simulink model "FOC_sensored"  (R2026a)
settings: Solver=VariableStepAuto  StopTime=0.5  MaxStep=1e-4  RelTol=1e-4
values from neighbouring files (symbols this model uses):
  Encoder_resolution = 4000    [FOC_sensored_script.m]
  In = 1    [FOC_sensored_script.m]
  J = 0.1e-4    (= 1e-05)    [FOC_sensored_script.m]
  Kr_cont_current = (2*omega_n*tau_q*zeta - 1) / K_q    [FOC_sensored_script.m]
  Kr_cont_speed = (2*omega_n_speed*tau_w*zeta_speed - 1) / K_w    [FOC_sensored_script.m]
  Kr_direct_back_current = (1-delta2*exp(Ts_current/tau_q)) / (K_q*(exp(Ts_current/tau_q)-1))    [FOC_sensored_script.m]
  Kr_direct_back_speed = (1-delta2*exp(Ts_speed/tau_w)) / (K_w*(exp(Ts_speed/tau_w)-1))    [FOC_sensored_script.m]
  Kr_direct_forw_current = (1+(1+delta1)*exp(Ts_current/tau_q)) / (K_q*(exp(Ts_current/tau_q)-1))    [FOC_sensored_script.m]
  Kr_direct_tustin_current = (2-exp(Ts_current/tau_q)*(delta2-delta1-1)) / (2*K_q*(exp(Ts_current/tau_q)-1))    [FOC_sensored_script.m]
  Kr_direct_tustin_speed = (2-exp(Ts_speed/tau_w)*(delta2-delta1-1)) / (2*K_w*(exp(Ts_speed/tau_w)-1))    [FOC_sensored_script.m]
  Ls = 330e-6/2    (= 0.000165)    [FOC_sensored_script.m]
  Mn = Pn/wn    [FOC_sensored_script.m]
  nn = ns/pp    (= 6000)    [FOC_sensored_script.m]
  pp = (60*fs)/ns    (= 4)    [FOC_sensored_script.m]
  Psir = 0.0064    [FOC_sensored_script.m]
  T_speed_feedback = 0.0005    [FOC_sensored_script.m]
  Ti_cont_current = (2*omega_n*tau_q*zeta - 1) / (tau_q * omega_n^2)    [FOC_sensored_script.m]
  Ti_cont_speed = (2*omega_n_speed*tau_w*zeta_speed - 1) / (tau_w * omega_n_speed^2)    [FOC_sensored_script.m]
  Ti_direct_back_current = Ts_current * (exp(-Ts_current/tau_q)-delta2) / (1+delta1+delta2)    [FOC_sensored_script.m]
  Ti_direct_back_speed = Ts_speed * (exp(-Ts_speed/tau_w)-delta2) / (1+delta1+delta2)    [FOC_sensored_script.m]
  Ti_direct_forw_current = Ts_current * (1+delta1+exp(-Ts_current/tau_q)) / (1+delta1+delta2)    [FOC_sensored_script.m]
  Ti_direct_forw_speed = Ts_speed * (1+delta1+exp(-Ts_speed/tau_w)) / (1+delta1+delta2)    [FOC_sensored_script.m]
  Ti_direct_tustin_current = Ts_current*(2*exp(-Ts_current/tau_q)+delta1-delta2+1) / (2*(1+delta1+delta2))    [FOC_sensored_script.m]
  Ti_direct_tustin_speed = Ts_speed*(2*exp(-Ts_speed/tau_w)+delta1-delta2+1) / (2*(1+delta1+delta2))    [FOC_sensored_script.m]
  Ts_current = 100e-6    (= 0.0001)    [FOC_sensored_script.m]
  Udc = 24    [FOC_sensored_script.m]
undefined symbols (not defined in the file or in its folder): Ld, Lq
libraries: fl_lib x48, nesl_utility x42, ee_lib x18, eeTransforms x12
(part 2 of 3)

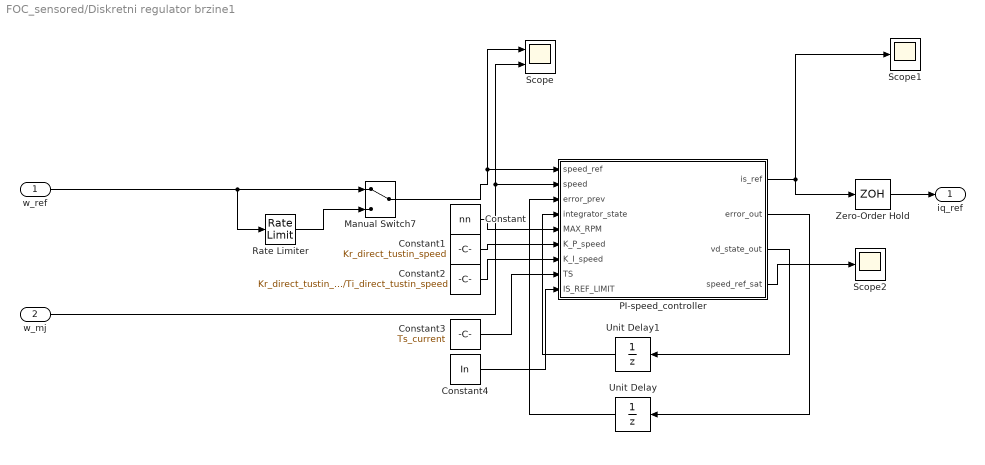
== system FOC_sensored/Diskretni regulator brzine1 ==
  w_ref : Inport
  w_mj : Inport  Port=2
  Constant : Constant  Value=nn  SampleTime=Ts_current
  Constant1 : Constant  Value=Kr_direct_tustin_speed  SampleTime=Ts_current
  Constant2 : Constant  Value=Kr_direct_tustin_speed/Ti_direct_tustin_speed  SampleTime=Ts_current
  Constant3 : Constant  Value=Ts_current  SampleTime=Ts_current
  Constant4 : Constant  Value=In  SampleTime=Ts_current
  Manual Switch7 : ManualSwitch
  PI-speed_controller : MATLAB Function  TreatAsAtomicUnit=on
  Rate Limiter : RateLimiter  RisingSlewLimit=Mn/J  FallingSlewLimit=-Mn/J  SampleTimeMode=inherited
  Scope : Scope  NumInputPorts=2
      settings: ActiveDisplayYMinimum=-62.500309400179823  ActiveDisplayYMaximum=562.50278460161849  DataLoggingVariableName=ScopeData4
  Scope1 : Scope
      settings: ActiveDisplayYMinimum=-62.5113191756852  ActiveDisplayYMaximum=70.802739564965421  DataLoggingVariableName=ScopeData5
  Scope2 : Scope
      settings: ActiveDisplayYMinimum=-1  ActiveDisplayYMaximum=1  DataLoggingVariableName=ScopeData10
  Unit Delay : UnitDelay  SampleTime=Ts_current
  Unit Delay1 : UnitDelay  SampleTime=Ts_current
  Zero-Order Hold : ZeroOrderHold  SampleTime=Ts_current
  iq_ref : Outport
  wires:
  Rate Limiter/1 -> Manual Switch7/2
  PI-speed_controller/2(error_out) -> Unit Delay/1
  Unit Delay/1 -> PI-speed_controller/3(error_prev)
  PI-speed_controller/3(vd_state_out) -> Unit Delay1/1
  Unit Delay1/1 -> PI-speed_controller/4(integrator_state)
  w_ref/1 -> Manual Switch7/1, Rate Limiter/1
  Manual Switch7/1 -> Scope/1, PI-speed_controller/1(speed_ref)
  w_mj/1 -> Scope/2, PI-speed_controller/2(speed)
  PI-speed_controller/1(is_ref) -> Scope1/1, Zero-Order Hold/1
  PI-speed_controller/4(speed_ref_sat) -> Scope2/1
  Zero-Order Hold/1 -> iq_ref/1
  Constant/1 -> PI-speed_controller/5(MAX_RPM)
  Constant1/1 -> PI-speed_controller/6(K_P_speed)
  Constant2/1 -> PI-speed_controller/7(K_I_speed)
  Constant3/1 -> PI-speed_controller/8(TS)
  Constant4/1 -> PI-speed_controller/9(IS_REF_LIMIT)

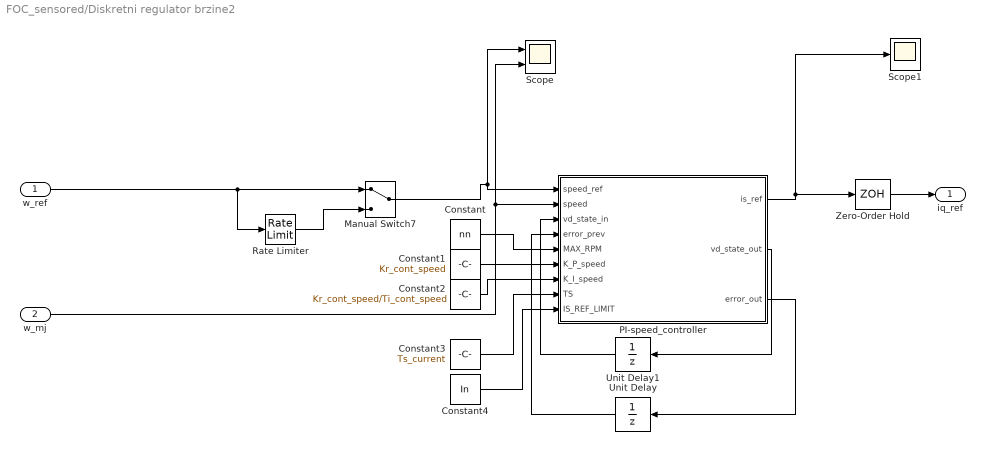
== system FOC_sensored/Diskretni regulator brzine2 ==
  w_ref : Inport
  w_mj : Inport  Port=2
  Constant : Constant  Value=nn  SampleTime=Ts_current
  Constant1 : Constant  Value=Kr_cont_speed  SampleTime=Ts_current
  Constant2 : Constant  Value=Kr_cont_speed/Ti_cont_speed  SampleTime=Ts_current
  Constant3 : Constant  Value=Ts_current  SampleTime=Ts_current
  Constant4 : Constant  Value=In  SampleTime=Ts_current
  Manual Switch7 : ManualSwitch
  PI-speed_controller : MATLAB Function  TreatAsAtomicUnit=on
  Rate Limiter : RateLimiter  RisingSlewLimit=Mn/J  FallingSlewLimit=-Mn/J  SampleTimeMode=inherited
  Scope : Scope  NumInputPorts=2
      settings: ActiveDisplayYMinimum=-62.500309400179823  ActiveDisplayYMaximum=562.50278460161849  DataLoggingVariableName=ScopeData4
  Scope1 : Scope
      settings: ActiveDisplayYMinimum=-62.5113191756852  ActiveDisplayYMaximum=70.802739564965421  DataLoggingVariableName=ScopeData5
  Unit Delay : UnitDelay  SampleTime=Ts_current
  Unit Delay1 : UnitDelay  SampleTime=Ts_current
  Zero-Order Hold : ZeroOrderHold  SampleTime=Ts_current
  iq_ref : Outport
  wires:
  Rate Limiter/1 -> Manual Switch7/2
  PI-speed_controller/3(error_out) -> Unit Delay/1
  Unit Delay/1 -> PI-speed_controller/4(error_prev)
  PI-speed_controller/2(vd_state_out) -> Unit Delay1/1
  Unit Delay1/1 -> PI-speed_controller/3(vd_state_in)
  w_ref/1 -> Manual Switch7/1, Rate Limiter/1
  Manual Switch7/1 -> Scope/1, PI-speed_controller/1(speed_ref)
  w_mj/1 -> Scope/2, PI-speed_controller/2(speed)
  PI-speed_controller/1(is_ref) -> Scope1/1, Zero-Order Hold/1
  Zero-Order Hold/1 -> iq_ref/1
  Constant/1 -> PI-speed_controller/5(MAX_RPM)
  Constant1/1 -> PI-speed_controller/6(K_P_speed)
  Constant2/1 -> PI-speed_controller/7(K_I_speed)
  Constant3/1 -> PI-speed_controller/8(TS)
  Constant4/1 -> PI-speed_controller/9(IS_REF_LIMIT)

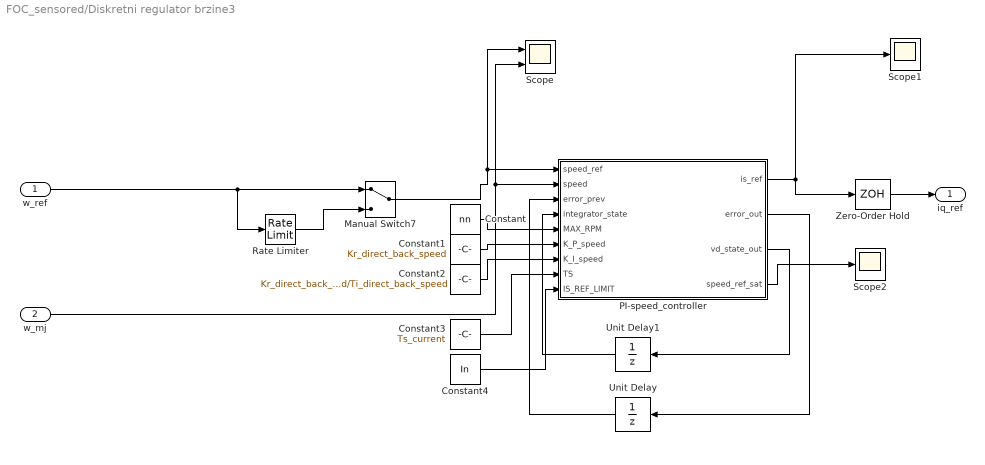
== system FOC_sensored/Diskretni regulator brzine3 ==
  w_ref : Inport
  w_mj : Inport  Port=2
  Constant : Constant  Value=nn  SampleTime=Ts_current
  Constant1 : Constant  Value=Kr_direct_back_speed  SampleTime=Ts_current
  Constant2 : Constant  Value=Kr_direct_back_speed/Ti_direct_back_speed  SampleTime=Ts_current
  Constant3 : Constant  Value=Ts_current  SampleTime=Ts_current
  Constant4 : Constant  Value=In  SampleTime=Ts_current
  Manual Switch7 : ManualSwitch
  PI-speed_controller : MATLAB Function  TreatAsAtomicUnit=on
  Rate Limiter : RateLimiter  RisingSlewLimit=Mn/J  FallingSlewLimit=-Mn/J  SampleTimeMode=inherited
  Scope : Scope  NumInputPorts=2
      settings: ActiveDisplayYMinimum=-62.500309400179823  ActiveDisplayYMaximum=562.50278460161849  DataLoggingVariableName=ScopeData4
  Scope1 : Scope
      settings: ActiveDisplayYMinimum=-62.5113191756852  ActiveDisplayYMaximum=70.802739564965421  DataLoggingVariableName=ScopeData5
  Scope2 : Scope
      settings: ActiveDisplayYMinimum=-1  ActiveDisplayYMaximum=1  DataLoggingVariableName=ScopeData10
  Unit Delay : UnitDelay  SampleTime=Ts_current
  Unit Delay1 : UnitDelay  SampleTime=Ts_current
  Zero-Order Hold : ZeroOrderHold  SampleTime=Ts_current
  iq_ref : Outport
  wires:
  Rate Limiter/1 -> Manual Switch7/2
  PI-speed_controller/2(error_out) -> Unit Delay/1
  Unit Delay/1 -> PI-speed_controller/3(error_prev)
  PI-speed_controller/3(vd_state_out) -> Unit Delay1/1
  Unit Delay1/1 -> PI-speed_controller/4(integrator_state)
  w_ref/1 -> Manual Switch7/1, Rate Limiter/1
  Manual Switch7/1 -> Scope/1, PI-speed_controller/1(speed_ref)
  w_mj/1 -> Scope/2, PI-speed_controller/2(speed)
  PI-speed_controller/1(is_ref) -> Scope1/1, Zero-Order Hold/1
  PI-speed_controller/4(speed_ref_sat) -> Scope2/1
  Zero-Order Hold/1 -> iq_ref/1
  Constant/1 -> PI-speed_controller/5(MAX_RPM)
  Constant1/1 -> PI-speed_controller/6(K_P_speed)
  Constant2/1 -> PI-speed_controller/7(K_I_speed)
  Constant3/1 -> PI-speed_controller/8(TS)
  Constant4/1 -> PI-speed_controller/9(IS_REF_LIMIT)

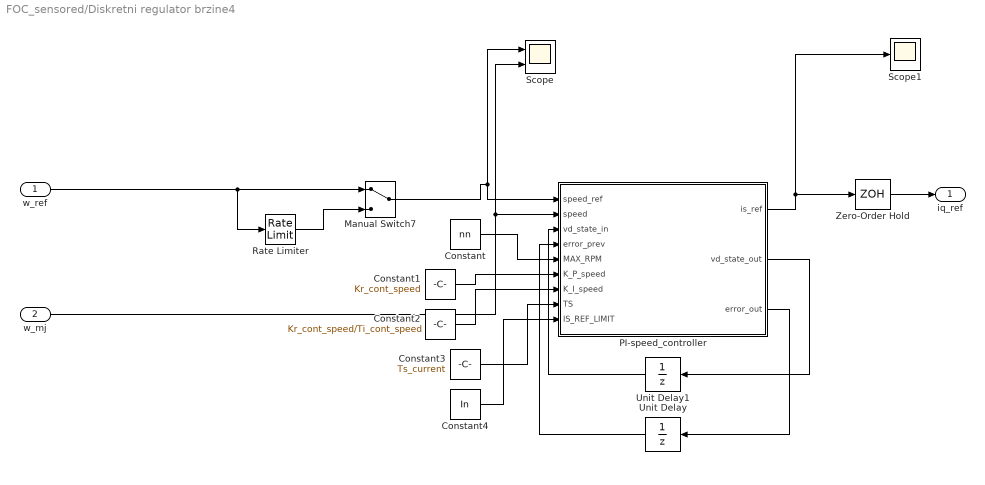
== system FOC_sensored/Diskretni regulator brzine4 ==
  w_ref : Inport
  w_mj : Inport  Port=2
  Constant : Constant  Value=nn  SampleTime=Ts_current
  Constant1 : Constant  Value=Kr_cont_speed  SampleTime=Ts_current
  Constant2 : Constant  Value=Kr_cont_speed/Ti_cont_speed  SampleTime=Ts_current
  Constant3 : Constant  Value=Ts_current  SampleTime=Ts_current
  Constant4 : Constant  Value=In  SampleTime=Ts_current
  Manual Switch7 : ManualSwitch
  PI-speed_controller : MATLAB Function  TreatAsAtomicUnit=on
  Rate Limiter : RateLimiter  RisingSlewLimit=Mn/J  FallingSlewLimit=-Mn/J  SampleTimeMode=inherited
  Scope : Scope  NumInputPorts=2
      settings: ActiveDisplayYMinimum=-62.500309400179823  ActiveDisplayYMaximum=562.50278460161849  DataLoggingVariableName=ScopeData4
  Scope1 : Scope
      settings: ActiveDisplayYMinimum=-62.5113191756852  ActiveDisplayYMaximum=70.802739564965421  DataLoggingVariableName=ScopeData5
  Unit Delay : UnitDelay  SampleTime=Ts_current
  Unit Delay1 : UnitDelay  SampleTime=Ts_current
  Zero-Order Hold : ZeroOrderHold  SampleTime=Ts_current
  iq_ref : Outport
  wires:
  Rate Limiter/1 -> Manual Switch7/2
  PI-speed_controller/3(error_out) -> Unit Delay/1
  Unit Delay/1 -> PI-speed_controller/4(error_prev)
  PI-speed_controller/2(vd_state_out) -> Unit Delay1/1
  Unit Delay1/1 -> PI-speed_controller/3(vd_state_in)
  w_ref/1 -> Manual Switch7/1, Rate Limiter/1
  Manual Switch7/1 -> Scope/1, PI-speed_controller/1(speed_ref)
  w_mj/1 -> Scope/2, PI-speed_controller/2(speed)
  PI-speed_controller/1(is_ref) -> Scope1/1, Zero-Order Hold/1
  Zero-Order Hold/1 -> iq_ref/1
  Constant/1 -> PI-speed_controller/5(MAX_RPM)
  Constant1/1 -> PI-speed_controller/6(K_P_speed)
  Constant2/1 -> PI-speed_controller/7(K_I_speed)
  Constant3/1 -> PI-speed_controller/8(TS)
  Constant4/1 -> PI-speed_controller/9(IS_REF_LIMIT)

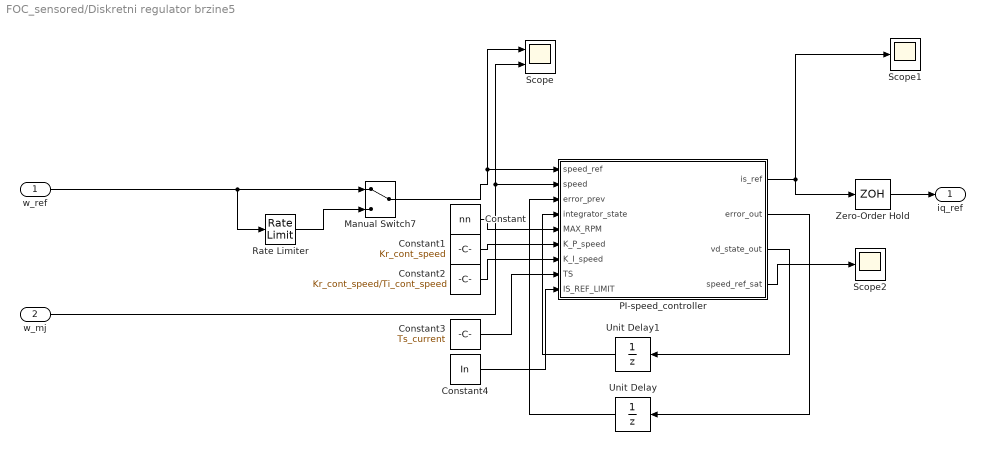
== system FOC_sensored/Diskretni regulator brzine5 ==
  w_ref : Inport
  w_mj : Inport  Port=2
  Constant : Constant  Value=nn  SampleTime=Ts_current
  Constant1 : Constant  Value=Kr_cont_speed  SampleTime=Ts_current
  Constant2 : Constant  Value=Kr_cont_speed/Ti_cont_speed  SampleTime=Ts_current
  Constant3 : Constant  Value=Ts_current  SampleTime=Ts_current
  Constant4 : Constant  Value=In  SampleTime=Ts_current
  Manual Switch7 : ManualSwitch
  PI-speed_controller : MATLAB Function  TreatAsAtomicUnit=on
  Rate Limiter : RateLimiter  RisingSlewLimit=Mn/J  FallingSlewLimit=-Mn/J  SampleTimeMode=inherited
  Scope : Scope  NumInputPorts=2
      settings: ActiveDisplayYMinimum=-62.500309400179823  ActiveDisplayYMaximum=562.50278460161849  DataLoggingVariableName=ScopeData4
  Scope1 : Scope
      settings: ActiveDisplayYMinimum=-62.5113191756852  ActiveDisplayYMaximum=70.802739564965421  DataLoggingVariableName=ScopeData5
  Scope2 : Scope
      settings: ActiveDisplayYMinimum=-1  ActiveDisplayYMaximum=1  DataLoggingVariableName=ScopeData10
  Unit Delay : UnitDelay  SampleTime=Ts_current
  Unit Delay1 : UnitDelay  SampleTime=Ts_current
  Zero-Order Hold : ZeroOrderHold  SampleTime=Ts_current
  iq_ref : Outport
  wires:
  Rate Limiter/1 -> Manual Switch7/2
  PI-speed_controller/2(error_out) -> Unit Delay/1
  Unit Delay/1 -> PI-speed_controller/3(error_prev)
  PI-speed_controller/3(vd_state_out) -> Unit Delay1/1
  Unit Delay1/1 -> PI-speed_controller/4(integrator_state)
  w_ref/1 -> Manual Switch7/1, Rate Limiter/1
  Manual Switch7/1 -> Scope/1, PI-speed_controller/1(speed_ref)
  w_mj/1 -> Scope/2, PI-speed_controller/2(speed)
  PI-speed_controller/1(is_ref) -> Scope1/1, Zero-Order Hold/1
  PI-speed_controller/4(speed_ref_sat) -> Scope2/1
  Zero-Order Hold/1 -> iq_ref/1
  Constant/1 -> PI-speed_controller/5(MAX_RPM)
  Constant1/1 -> PI-speed_controller/6(K_P_speed)
  Constant2/1 -> PI-speed_controller/7(K_I_speed)
  Constant3/1 -> PI-speed_controller/8(TS)
  Constant4/1 -> PI-speed_controller/9(IS_REF_LIMIT)

== system FOC_sensored/Diskretni regulator brzine6 ==
  w_ref : Inport
  w_mj : Inport  Port=2
  Constant : Constant  Value=nn  SampleTime=Ts_current
  Constant1 : Constant  Value=Kr_cont_speed  SampleTime=Ts_current
  Constant2 : Constant  Value=Kr_cont_speed/Ti_cont_speed  SampleTime=Ts_current
  Constant3 : Constant  Value=Ts_current  SampleTime=Ts_current
  Constant4 : Constant  Value=In  SampleTime=Ts_current
  Manual Switch7 : ManualSwitch
  PI-speed_controller : MATLAB Function  TreatAsAtomicUnit=on
  Rate Limiter : RateLimiter  RisingSlewLimit=Mn/J  FallingSlewLimit=-Mn/J  SampleTimeMode=inherited
  Scope : Scope  NumInputPorts=2
      settings: ActiveDisplayYMinimum=-62.500309400179823  ActiveDisplayYMaximum=562.50278460161849  DataLoggingVariableName=ScopeData4
  Scope1 : Scope
      settings: ActiveDisplayYMinimum=-62.5113191756852  ActiveDisplayYMaximum=70.802739564965421  DataLoggingVariableName=ScopeData5
  Unit Delay : UnitDelay  SampleTime=Ts_current
  Unit Delay1 : UnitDelay  SampleTime=Ts_current
  Zero-Order Hold : ZeroOrderHold  SampleTime=Ts_current
  iq_ref : Outport
  wires:
  Rate Limiter/1 -> Manual Switch7/2
  PI-speed_controller/3(error_out) -> Unit Delay/1
  Unit Delay/1 -> PI-speed_controller/4(error_prev)
  PI-speed_controller/2(vd_state_out) -> Unit Delay1/1
  Unit Delay1/1 -> PI-speed_controller/3(vd_state_in)
  w_ref/1 -> Manual Switch7/1, Rate Limiter/1
  Manual Switch7/1 -> Scope/1, PI-speed_controller/1(speed_ref)
  w_mj/1 -> Scope/2, PI-speed_controller/2(speed)
  PI-speed_controller/1(is_ref) -> Scope1/1, Zero-Order Hold/1
  Zero-Order Hold/1 -> iq_ref/1
  Constant/1 -> PI-speed_controller/5(MAX_RPM)
  Constant1/1 -> PI-speed_controller/6(K_P_speed)
  Constant2/1 -> PI-speed_controller/7(K_I_speed)
  Constant3/1 -> PI-speed_controller/8(TS)
  Constant4/1 -> PI-speed_controller/9(IS_REF_LIMIT)

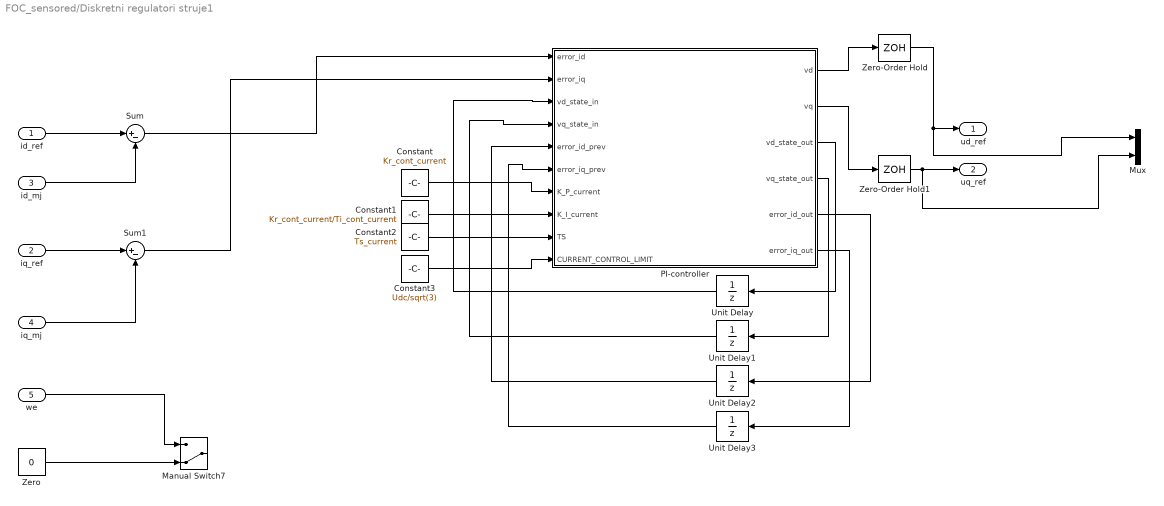
== system FOC_sensored/Diskretni regulatori struje1 ==
  id_ref : Inport
  iq_ref : Inport  Port=2
  id_mj : Inport  Port=3
  iq_mj : Inport  Port=4
  we : Inport  Port=5
  Constant : Constant  Value=Kr_cont_current  SampleTime=Ts_current
  Constant1 : Constant  Value=Kr_cont_current/Ti_cont_current  SampleTime=Ts_current
  Constant2 : Constant  Value=Ts_current  SampleTime=Ts_current
  Constant3 : Constant  Value=Udc/sqrt(3)  SampleTime=Ts_current
  Manual Switch7 : ManualSwitch  CurrentSetting=0
  Mux : Mux  Inputs=2
  PI-controller : MATLAB Function  TreatAsAtomicUnit=on
  Sum : Sum  Inputs=|+-
  Sum1 : Sum  Inputs=|+-
  Unit Delay{,1..3} (4 alike) : UnitDelay  SampleTime=Ts_current
  Zero : Constant  Value=0  OutDataTypeStr=Inherit: Inherit via back propagation
  Zero-Order Hold : ZeroOrderHold  SampleTime=Ts_current
  Zero-Order Hold1 : ZeroOrderHold  SampleTime=Ts_current
  ud_ref : Outport
  uq_ref : Outport  Port=2
  wires:
  id_ref/1 -> Sum/1
  iq_ref/1 -> Sum1/1
  Sum/1 -> PI-controller/1(error_id)
  id_mj/1 -> Sum/2
  iq_mj/1 -> Sum1/2
  PI-controller/3(vd_state_out) -> Unit Delay/1
  PI-controller/4(vq_state_out) -> Unit Delay1/1
  PI-controller/1(vd) -> Zero-Order Hold/1
  PI-controller/2(vq) -> Zero-Order Hold1/1
  Zero-Order Hold/1 -> Mux/1, ud_ref/1
  Zero-Order Hold1/1 -> Mux/2, uq_ref/1
  Zero/1 -> Manual Switch7/2
  we/1 -> Manual Switch7/1
  Sum1/1 -> PI-controller/2(error_iq)
  Unit Delay/1 -> PI-controller/3(vd_state_in)
  Unit Delay1/1 -> PI-controller/4(vq_state_in)
  PI-controller/5(error_id_out) -> Unit Delay2/1
  Unit Delay2/1 -> PI-controller/5(error_id_prev)
  PI-controller/6(error_iq_out) -> Unit Delay3/1
  Unit Delay3/1 -> PI-controller/6(error_iq_prev)
  Constant/1 -> PI-controller/7(K_P_current)
  Constant1/1 -> PI-controller/8(K_I_current)
  Constant2/1 -> PI-controller/9(TS)
  Constant3/1 -> PI-controller/10(CURRENT_CONTROL_LIMIT)

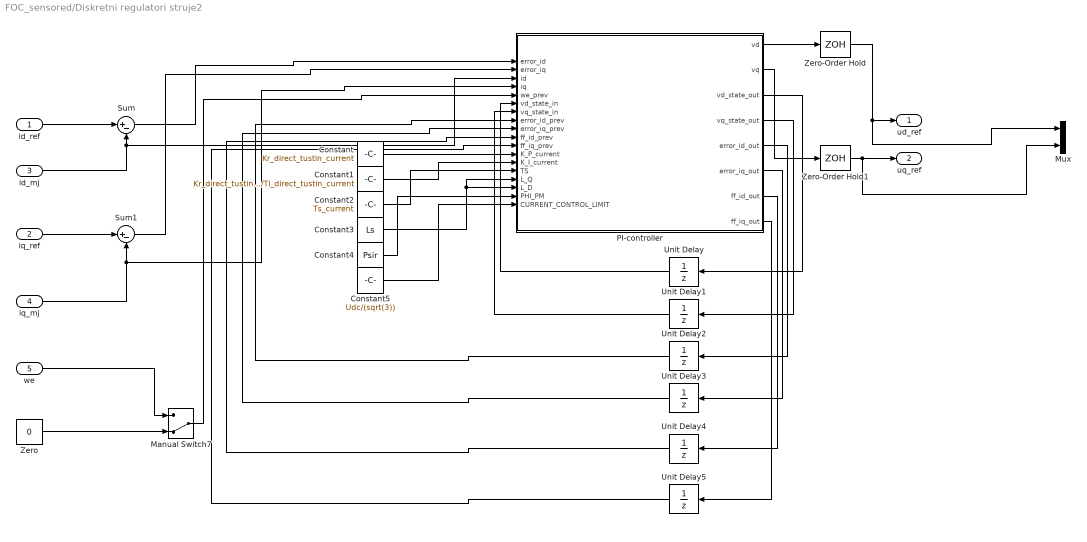
== system FOC_sensored/Diskretni regulatori struje2 ==
  id_ref : Inport
  iq_ref : Inport  Port=2
  id_mj : Inport  Port=3
  iq_mj : Inport  Port=4
  we : Inport  Port=5
  Constant : Constant  Value=Kr_direct_tustin_current  SampleTime=Ts_current
  Constant1 : Constant  Value=Kr_direct_tustin_current/Ti_direct_tustin_current  SampleTime=Ts_current
  Constant2 : Constant  Value=Ts_current  SampleTime=Ts_current
  Constant3 : Constant  Value=Ls  SampleTime=Ts_current
  Constant4 : Constant  Value=Psir  SampleTime=Ts_current
  Constant5 : Constant  Value=Udc/(sqrt(3))  SampleTime=Ts_current
  Manual Switch7 : ManualSwitch  CurrentSetting=0
  Mux : Mux  Inputs=2
  PI-controller : MATLAB Function  TreatAsAtomicUnit=on
  Sum : Sum  Inputs=|+-
  Sum1 : Sum  Inputs=|+-
  Unit Delay{,1..5} (6 alike) : UnitDelay  SampleTime=Ts_current
  Zero : Constant  Value=0  OutDataTypeStr=Inherit: Inherit via back propagation
  Zero-Order Hold : ZeroOrderHold  SampleTime=Ts_current
  Zero-Order Hold1 : ZeroOrderHold  SampleTime=Ts_current
  ud_ref : Outport
  uq_ref : Outport  Port=2
  wires:
  id_ref/1 -> Sum/1
  iq_ref/1 -> Sum1/1
  Sum/1 -> PI-controller/1(error_id)
  Sum1/1 -> PI-controller/2(error_iq)
  id_mj/1 -> Sum/2, PI-controller/3(id)
  iq_mj/1 -> PI-controller/4(iq), Sum1/2
  PI-controller/3(vd_state_out) -> Unit Delay/1
  PI-controller/4(vq_state_out) -> Unit Delay1/1
  PI-controller/5(error_id_out) -> Unit Delay2/1
  PI-controller/6(error_iq_out) -> Unit Delay3/1
  Unit Delay/1 -> PI-controller/6(vd_state_in)
  Unit Delay1/1 -> PI-controller/7(vq_state_in)
  Unit Delay2/1 -> PI-controller/8(error_id_prev)
  Unit Delay3/1 -> PI-controller/9(error_iq_prev)
  PI-controller/1(vd) -> Zero-Order Hold/1
  PI-controller/2(vq) -> Zero-Order Hold1/1
  Zero-Order Hold/1 -> Mux/1, ud_ref/1
  Zero-Order Hold1/1 -> Mux/2, uq_ref/1
  PI-controller/7(ff_id_out) -> Unit Delay4/1
  PI-controller/8(ff_iq_out) -> Unit Delay5/1
  Unit Delay4/1 -> PI-controller/10(ff_id_prev)
  Unit Delay5/1 -> PI-controller/11(ff_iq_prev)
  Zero/1 -> Manual Switch7/2
  Manual Switch7/1 -> PI-controller/5(we_prev)
  we/1 -> Manual Switch7/1
  Constant/1 -> PI-controller/12(K_P_current)
  Constant1/1 -> PI-controller/13(K_I_current)
  Constant2/1 -> PI-controller/14(TS)
  Constant3/1 -> PI-controller/16(L_D), PI-controller/15(L_Q)
  Constant4/1 -> PI-controller/17(PHI_PM)
  Constant5/1 -> PI-controller/18(CURRENT_CONTROL_LIMIT)

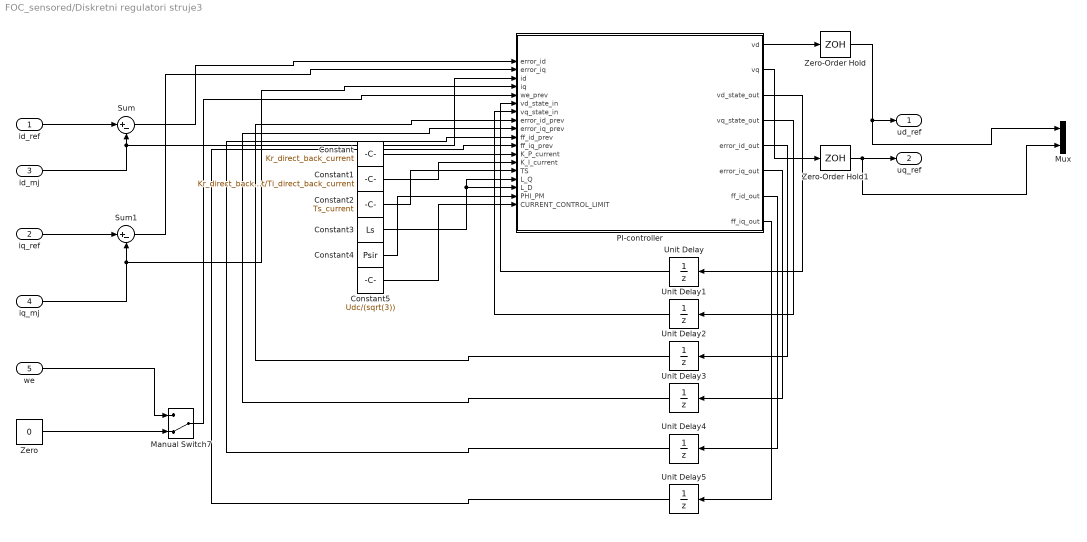
== system FOC_sensored/Diskretni regulatori struje3 ==
  id_ref : Inport
  iq_ref : Inport  Port=2
  id_mj : Inport  Port=3
  iq_mj : Inport  Port=4
  we : Inport  Port=5
  Constant : Constant  Value=Kr_direct_back_current  SampleTime=Ts_current
  Constant1 : Constant  Value=Kr_direct_back_current/Ti_direct_back_current  SampleTime=Ts_current
  Constant2 : Constant  Value=Ts_current  SampleTime=Ts_current
  Constant3 : Constant  Value=Ls  SampleTime=Ts_current
  Constant4 : Constant  Value=Psir  SampleTime=Ts_current
  Constant5 : Constant  Value=Udc/(sqrt(3))  SampleTime=Ts_current
  Manual Switch7 : ManualSwitch  CurrentSetting=0
  Mux : Mux  Inputs=2
  PI-controller : MATLAB Function  TreatAsAtomicUnit=on
  Sum : Sum  Inputs=|+-
  Sum1 : Sum  Inputs=|+-
  Unit Delay{,1..5} (6 alike) : UnitDelay  SampleTime=Ts_current
  Zero : Constant  Value=0  OutDataTypeStr=Inherit: Inherit via back propagation
  Zero-Order Hold : ZeroOrderHold  SampleTime=Ts_current
  Zero-Order Hold1 : ZeroOrderHold  SampleTime=Ts_current
  ud_ref : Outport
  uq_ref : Outport  Port=2
  wires:
  id_ref/1 -> Sum/1
  iq_ref/1 -> Sum1/1
  Sum/1 -> PI-controller/1(error_id)
  Sum1/1 -> PI-controller/2(error_iq)
  id_mj/1 -> Sum/2, PI-controller/3(id)
  iq_mj/1 -> PI-controller/4(iq), Sum1/2
  PI-controller/3(vd_state_out) -> Unit Delay/1
  PI-controller/4(vq_state_out) -> Unit Delay1/1
  PI-controller/5(error_id_out) -> Unit Delay2/1
  PI-controller/6(error_iq_out) -> Unit Delay3/1
  Unit Delay/1 -> PI-controller/6(vd_state_in)
  Unit Delay1/1 -> PI-controller/7(vq_state_in)
  Unit Delay2/1 -> PI-controller/8(error_id_prev)
  Unit Delay3/1 -> PI-controller/9(error_iq_prev)
  PI-controller/1(vd) -> Zero-Order Hold/1
  PI-controller/2(vq) -> Zero-Order Hold1/1
  Zero-Order Hold/1 -> Mux/1, ud_ref/1
  Zero-Order Hold1/1 -> Mux/2, uq_ref/1
  PI-controller/7(ff_id_out) -> Unit Delay4/1
  PI-controller/8(ff_iq_out) -> Unit Delay5/1
  Unit Delay4/1 -> PI-controller/10(ff_id_prev)
  Unit Delay5/1 -> PI-controller/11(ff_iq_prev)
  Zero/1 -> Manual Switch7/2
  Manual Switch7/1 -> PI-controller/5(we_prev)
  we/1 -> Manual Switch7/1
  Constant/1 -> PI-controller/12(K_P_current)
  Constant1/1 -> PI-controller/13(K_I_current)
  Constant2/1 -> PI-controller/14(TS)
  Constant3/1 -> PI-controller/16(L_D), PI-controller/15(L_Q)
  Constant4/1 -> PI-controller/17(PHI_PM)
  Constant5/1 -> PI-controller/18(CURRENT_CONTROL_LIMIT)

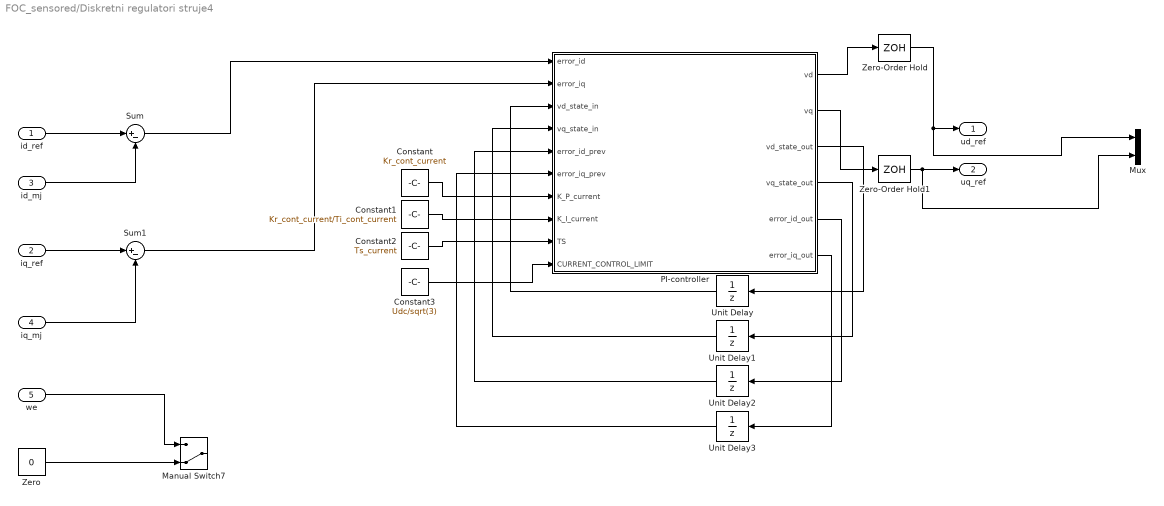
== system FOC_sensored/Diskretni regulatori struje4 ==
  id_ref : Inport
  iq_ref : Inport  Port=2
  id_mj : Inport  Port=3
  iq_mj : Inport  Port=4
  we : Inport  Port=5
  Constant : Constant  Value=Kr_cont_current  SampleTime=Ts_current
  Constant1 : Constant  Value=Kr_cont_current/Ti_cont_current  SampleTime=Ts_current
  Constant2 : Constant  Value=Ts_current  SampleTime=Ts_current
  Constant3 : Constant  Value=Udc/sqrt(3)  SampleTime=Ts_current
  Manual Switch7 : ManualSwitch  CurrentSetting=0
  Mux : Mux  Inputs=2
  PI-controller : MATLAB Function  TreatAsAtomicUnit=on
  Sum : Sum  Inputs=|+-
  Sum1 : Sum  Inputs=|+-
  Unit Delay{,1..3} (4 alike) : UnitDelay  SampleTime=Ts_current
  Zero : Constant  Value=0  OutDataTypeStr=Inherit: Inherit via back propagation
  Zero-Order Hold : ZeroOrderHold  SampleTime=Ts_current
  Zero-Order Hold1 : ZeroOrderHold  SampleTime=Ts_current
  ud_ref : Outport
  uq_ref : Outport  Port=2
  wires:
  id_ref/1 -> Sum/1
  iq_ref/1 -> Sum1/1
  Sum/1 -> PI-controller/1(error_id)
  id_mj/1 -> Sum/2
  iq_mj/1 -> Sum1/2
  PI-controller/3(vd_state_out) -> Unit Delay/1
  PI-controller/4(vq_state_out) -> Unit Delay1/1
  PI-controller/1(vd) -> Zero-Order Hold/1
  PI-controller/2(vq) -> Zero-Order Hold1/1
  Zero-Order Hold/1 -> Mux/1, ud_ref/1
  Zero-Order Hold1/1 -> Mux/2, uq_ref/1
  Zero/1 -> Manual Switch7/2
  we/1 -> Manual Switch7/1
  Sum1/1 -> PI-controller/2(error_iq)
  Unit Delay/1 -> PI-controller/3(vd_state_in)
  Unit Delay1/1 -> PI-controller/4(vq_state_in)
  PI-controller/5(error_id_out) -> Unit Delay2/1
  Unit Delay2/1 -> PI-controller/5(error_id_prev)
  PI-controller/6(error_iq_out) -> Unit Delay3/1
  Unit Delay3/1 -> PI-controller/6(error_iq_prev)
  Constant/1 -> PI-controller/7(K_P_current)
  Constant1/1 -> PI-controller/8(K_I_current)
  Constant2/1 -> PI-controller/9(TS)
  Constant3/1 -> PI-controller/10(CURRENT_CONTROL_LIMIT)

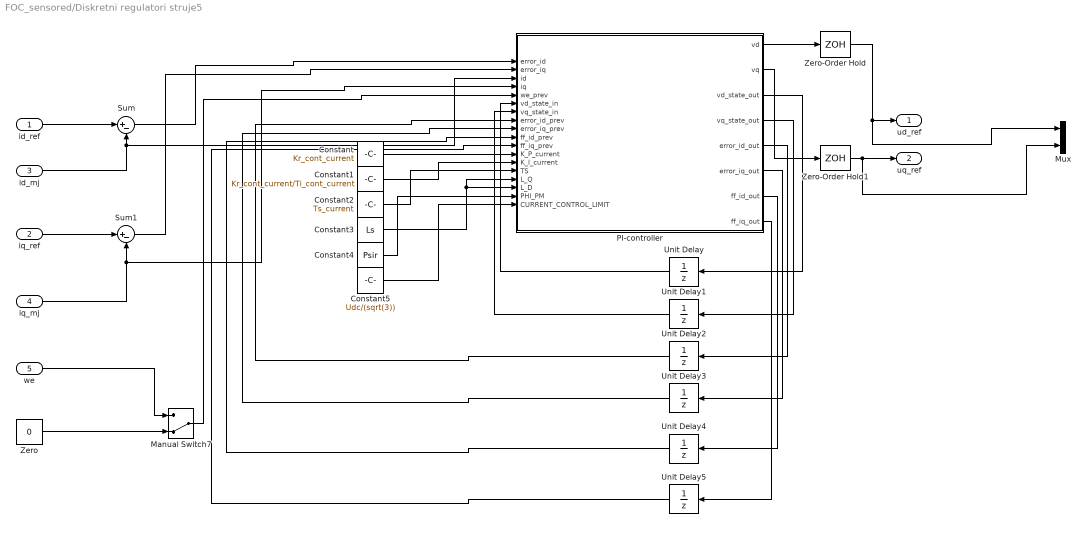
== system FOC_sensored/Diskretni regulatori struje5 ==
  id_ref : Inport
  iq_ref : Inport  Port=2
  id_mj : Inport  Port=3
  iq_mj : Inport  Port=4
  we : Inport  Port=5
  Constant : Constant  Value=Kr_cont_current  SampleTime=Ts_current
  Constant1 : Constant  Value=Kr_cont_current/Ti_cont_current  SampleTime=Ts_current
  Constant2 : Constant  Value=Ts_current  SampleTime=Ts_current
  Constant3 : Constant  Value=Ls  SampleTime=Ts_current
  Constant4 : Constant  Value=Psir  SampleTime=Ts_current
  Constant5 : Constant  Value=Udc/(sqrt(3))  SampleTime=Ts_current
  Manual Switch7 : ManualSwitch  CurrentSetting=0
  Mux : Mux  Inputs=2
  PI-controller : MATLAB Function  TreatAsAtomicUnit=on
  Sum : Sum  Inputs=|+-
  Sum1 : Sum  Inputs=|+-
  Unit Delay{,1..5} (6 alike) : UnitDelay  SampleTime=Ts_current
  Zero : Constant  Value=0  OutDataTypeStr=Inherit: Inherit via back propagation
  Zero-Order Hold : ZeroOrderHold  SampleTime=Ts_current
  Zero-Order Hold1 : ZeroOrderHold  SampleTime=Ts_current
  ud_ref : Outport
  uq_ref : Outport  Port=2
  wires:
  id_ref/1 -> Sum/1
  iq_ref/1 -> Sum1/1
  Sum/1 -> PI-controller/1(error_id)
  Sum1/1 -> PI-controller/2(error_iq)
  id_mj/1 -> Sum/2, PI-controller/3(id)
  iq_mj/1 -> PI-controller/4(iq), Sum1/2
  PI-controller/3(vd_state_out) -> Unit Delay/1
  PI-controller/4(vq_state_out) -> Unit Delay1/1
  PI-controller/5(error_id_out) -> Unit Delay2/1
  PI-controller/6(error_iq_out) -> Unit Delay3/1
  Unit Delay/1 -> PI-controller/6(vd_state_in)
  Unit Delay1/1 -> PI-controller/7(vq_state_in)
  Unit Delay2/1 -> PI-controller/8(error_id_prev)
  Unit Delay3/1 -> PI-controller/9(error_iq_prev)
  PI-controller/1(vd) -> Zero-Order Hold/1
  PI-controller/2(vq) -> Zero-Order Hold1/1
  Zero-Order Hold/1 -> Mux/1, ud_ref/1
  Zero-Order Hold1/1 -> Mux/2, uq_ref/1
  PI-controller/7(ff_id_out) -> Unit Delay4/1
  PI-controller/8(ff_iq_out) -> Unit Delay5/1
  Unit Delay4/1 -> PI-controller/10(ff_id_prev)
  Unit Delay5/1 -> PI-controller/11(ff_iq_prev)
  Zero/1 -> Manual Switch7/2
  Manual Switch7/1 -> PI-controller/5(we_prev)
  we/1 -> Manual Switch7/1
  Constant/1 -> PI-controller/12(K_P_current)
  Constant1/1 -> PI-controller/13(K_I_current)
  Constant2/1 -> PI-controller/14(TS)
  Constant3/1 -> PI-controller/16(L_D), PI-controller/15(L_Q)
  Constant4/1 -> PI-controller/17(PHI_PM)
  Constant5/1 -> PI-controller/18(CURRENT_CONTROL_LIMIT)

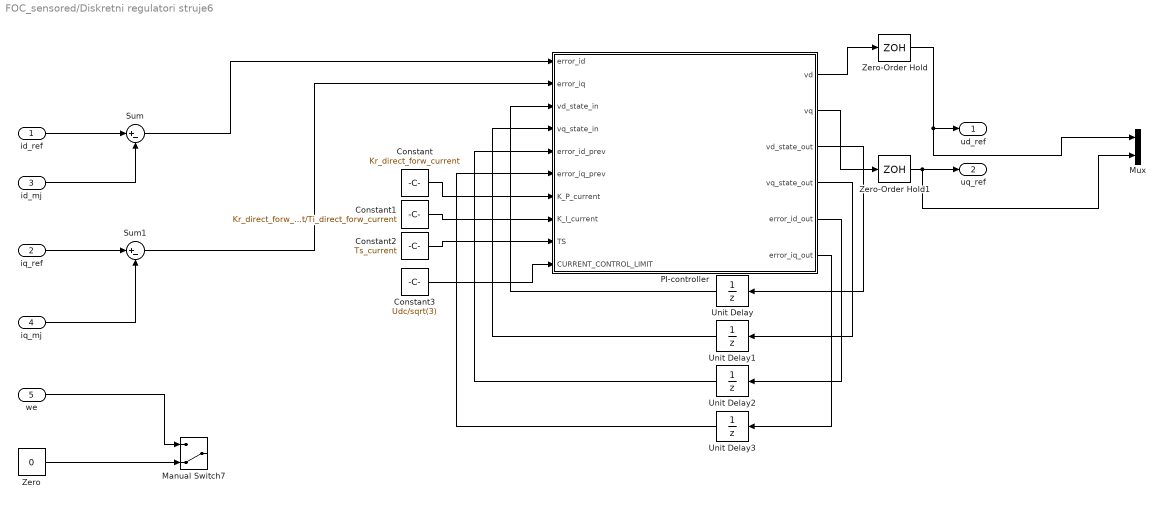
== system FOC_sensored/Diskretni regulatori struje6 ==
  id_ref : Inport
  iq_ref : Inport  Port=2
  id_mj : Inport  Port=3
  iq_mj : Inport  Port=4
  we : Inport  Port=5
  Constant : Constant  Value=Kr_direct_forw_current  SampleTime=Ts_current
  Constant1 : Constant  Value=Kr_direct_forw_current/Ti_direct_forw_current  SampleTime=Ts_current
  Constant2 : Constant  Value=Ts_current  SampleTime=Ts_current
  Constant3 : Constant  Value=Udc/sqrt(3)  SampleTime=Ts_current
  Manual Switch7 : ManualSwitch  CurrentSetting=0
  Mux : Mux  Inputs=2
  PI-controller : MATLAB Function  TreatAsAtomicUnit=on
  Sum : Sum  Inputs=|+-
  Sum1 : Sum  Inputs=|+-
  Unit Delay{,1..3} (4 alike) : UnitDelay  SampleTime=Ts_current
  Zero : Constant  Value=0  OutDataTypeStr=Inherit: Inherit via back propagation
  Zero-Order Hold : ZeroOrderHold  SampleTime=Ts_current
  Zero-Order Hold1 : ZeroOrderHold  SampleTime=Ts_current
  ud_ref : Outport
  uq_ref : Outport  Port=2
  wires:
  id_ref/1 -> Sum/1
  iq_ref/1 -> Sum1/1
  Sum/1 -> PI-controller/1(error_id)
  id_mj/1 -> Sum/2
  iq_mj/1 -> Sum1/2
  PI-controller/3(vd_state_out) -> Unit Delay/1
  PI-controller/4(vq_state_out) -> Unit Delay1/1
  PI-controller/1(vd) -> Zero-Order Hold/1
  PI-controller/2(vq) -> Zero-Order Hold1/1
  Zero-Order Hold/1 -> Mux/1, ud_ref/1
  Zero-Order Hold1/1 -> Mux/2, uq_ref/1
  Zero/1 -> Manual Switch7/2
  we/1 -> Manual Switch7/1
  Sum1/1 -> PI-controller/2(error_iq)
  Unit Delay/1 -> PI-controller/3(vd_state_in)
  Unit Delay1/1 -> PI-controller/4(vq_state_in)
  PI-controller/5(error_id_out) -> Unit Delay2/1
  Unit Delay2/1 -> PI-controller/5(error_id_prev)
  PI-controller/6(error_iq_out) -> Unit Delay3/1
  Unit Delay3/1 -> PI-controller/6(error_iq_prev)
  Constant/1 -> PI-controller/7(K_P_current)
  Constant1/1 -> PI-controller/8(K_I_current)
  Constant2/1 -> PI-controller/9(TS)
  Constant3/1 -> PI-controller/10(CURRENT_CONTROL_LIMIT)

== system FOC_sensored/Mjerenje momenta1 ==
  PS-Simulink Converter3 : nesl_utility/PS-Simulink Converter  PhysicalDomain=network_engine_domain  SubClassName=ps_output  LeftPortType=input  RightPortType=output  PseudoPeriodic=off  Frequencies=[]  VectorFormat=1-D array  Unit=N*m  AffineConversion=off
  Torque Sensor : fl_lib/Mechanical/Mechanical Sensors/Ideal Torque Sensor
  R : PMIOPort  Side=Left
  C : PMIOPort  Port=2  Side=Right
  Output : Outport
  wires:
  PS-Simulink Converter3/1 -> Output/1
  connections:
  Torque Sensor/RConn1 -- C/RConn1
  Torque Sensor/RConn2 -- PS-Simulink Converter3/LConn1
  Torque Sensor/LConn1 -- R/RConn1

== system FOC_sensored/Mjerenje momenta2 ==
  PS-Simulink Converter3 : nesl_utility/PS-Simulink Converter  PhysicalDomain=network_engine_domain  SubClassName=ps_output  LeftPortType=input  RightPortType=output  PseudoPeriodic=off  Frequencies=[]  VectorFormat=1-D array  Unit=N*m  AffineConversion=off
  Torque Sensor : fl_lib/Mechanical/Mechanical Sensors/Ideal Torque Sensor
  R : PMIOPort  Side=Left
  C : PMIOPort  Port=2  Side=Right
  Output : Outport
  wires:
  PS-Simulink Converter3/1 -> Output/1
  connections:
  Torque Sensor/RConn1 -- C/RConn1
  Torque Sensor/RConn2 -- PS-Simulink Converter3/LConn1
  Torque Sensor/LConn1 -- R/RConn1

== system FOC_sensored/Mjerenje momenta3 ==
  PS-Simulink Converter3 : nesl_utility/PS-Simulink Converter  PhysicalDomain=network_engine_domain  SubClassName=ps_output  LeftPortType=input  RightPortType=output  PseudoPeriodic=off  Frequencies=[]  VectorFormat=1-D array  Unit=N*m  AffineConversion=off
  Torque Sensor : fl_lib/Mechanical/Mechanical Sensors/Ideal Torque Sensor
  R : PMIOPort  Side=Left
  C : PMIOPort  Port=2  Side=Right
  Output : Outport
  wires:
  PS-Simulink Converter3/1 -> Output/1
  connections:
  Torque Sensor/RConn1 -- C/RConn1
  Torque Sensor/RConn2 -- PS-Simulink Converter3/LConn1
  Torque Sensor/LConn1 -- R/RConn1

== system FOC_sensored/Mjerenje momenta4 ==
  PS-Simulink Converter3 : nesl_utility/PS-Simulink Converter  PhysicalDomain=network_engine_domain  SubClassName=ps_output  LeftPortType=input  RightPortType=output  PseudoPeriodic=off  Frequencies=[]  VectorFormat=1-D array  Unit=N*m  AffineConversion=off
  Torque Sensor : fl_lib/Mechanical/Mechanical Sensors/Ideal Torque Sensor
  R : PMIOPort  Side=Left
  C : PMIOPort  Port=2  Side=Right
  Output : Outport
  wires:
  PS-Simulink Converter3/1 -> Output/1
  connections:
  Torque Sensor/RConn1 -- C/RConn1
  Torque Sensor/RConn2 -- PS-Simulink Converter3/LConn1
  Torque Sensor/LConn1 -- R/RConn1

== system FOC_sensored/Mjerenje momenta5 ==
  PS-Simulink Converter3 : nesl_utility/PS-Simulink Converter  PhysicalDomain=network_engine_domain  SubClassName=ps_output  LeftPortType=input  RightPortType=output  PseudoPeriodic=off  Frequencies=[]  VectorFormat=1-D array  Unit=N*m  AffineConversion=off
  Torque Sensor : fl_lib/Mechanical/Mechanical Sensors/Ideal Torque Sensor
  R : PMIOPort  Side=Left
  C : PMIOPort  Port=2  Side=Right
  Output : Outport
  wires:
  PS-Simulink Converter3/1 -> Output/1
  connections:
  Torque Sensor/RConn1 -- C/RConn1
  Torque Sensor/RConn2 -- PS-Simulink Converter3/LConn1
  Torque Sensor/LConn1 -- R/RConn1

== system FOC_sensored/Mjerenje momenta6 ==
  PS-Simulink Converter3 : nesl_utility/PS-Simulink Converter  PhysicalDomain=network_engine_domain  SubClassName=ps_output  LeftPortType=input  RightPortType=output  PseudoPeriodic=off  Frequencies=[]  VectorFormat=1-D array  Unit=N*m  AffineConversion=off
  Torque Sensor : fl_lib/Mechanical/Mechanical Sensors/Ideal Torque Sensor
  R : PMIOPort  Side=Left
  C : PMIOPort  Port=2  Side=Right
  Output : Outport
  wires:
  PS-Simulink Converter3/1 -> Output/1
  connections:
  Torque Sensor/RConn1 -- C/RConn1
  Torque Sensor/RConn2 -- PS-Simulink Converter3/LConn1
  Torque Sensor/LConn1 -- R/RConn1

== system FOC_sensored/Mjerenje kuta i brzine1 ==
  Constant4 : Constant  Value=2*pi
  Gain : Gain  Gain=pp
  Gain3 : Gain  Gain=pp
  MRRef : fl_lib/Mechanical/Rotational Elements/Mechanical Rotational Reference
  Math Function1 : Math  Operator=mod
  Motion Sensor : fl_lib/Mechanical/Mechanical Sensors/Ideal Rotational Motion Sensor  reference=foundation.enum.MeasurementReference.difference  acceleration_port=false  velocity_port=true  position_port=true  wrap_angle=simscape.enum.onoff.off  offset=0 deg
  PS-Simulink Converter1 : nesl_utility/PS-Simulink Converter  PhysicalDomain=network_engine_domain  SubClassName=ps_output  LeftPortType=input  RightPortType=output  PseudoPeriodic=off  Frequencies=[]  VectorFormat=1-D array  Unit=rad/s  AffineConversion=off
  PS-Simulink Converter2 : nesl_utility/PS-Simulink Converter  PhysicalDomain=network_engine_domain  SubClassName=ps_output  LeftPortType=input  RightPortType=output  PseudoPeriodic=off  Frequencies=[]  VectorFormat=1-D array  Unit=rad  AffineConversion=off
  R : PMIOPort  Side=Left
  we : Outport
  theta_e : Outport  Port=2
  wires:
  PS-Simulink Converter1/1 -> Gain/1
  Gain/1 -> we/1
  PS-Simulink Converter2/1 -> Gain3/1
  Constant4/1 -> Math Function1/2
  Gain3/1 -> Math Function1/1
  Math Function1/1 -> theta_e/1
  connections:
  R/RConn1 -- Motion Sensor/LConn1
  Motion Sensor/RConn2 -- PS-Simulink Converter1/LConn1
  MRRef/LConn1 -- Motion Sensor/RConn1
  Motion Sensor/RConn3 -- PS-Simulink Converter2/LConn1

== system FOC_sensored/Mjerenje kuta i brzine2 ==
  Constant4 : Constant  Value=2*pi
  Gain : Gain  Gain=pp
  Gain3 : Gain  Gain=pp
  MRRef : fl_lib/Mechanical/Rotational Elements/Mechanical Rotational Reference
  Math Function1 : Math  Operator=mod
  Motion Sensor : fl_lib/Mechanical/Mechanical Sensors/Ideal Rotational Motion Sensor  reference=foundation.enum.MeasurementReference.difference  acceleration_port=false  velocity_port=true  position_port=true  wrap_angle=simscape.enum.onoff.off  offset=0 deg
  PS-Simulink Converter1 : nesl_utility/PS-Simulink Converter  PhysicalDomain=network_engine_domain  SubClassName=ps_output  LeftPortType=input  RightPortType=output  PseudoPeriodic=off  Frequencies=[]  VectorFormat=1-D array  Unit=rad/s  AffineConversion=off
  PS-Simulink Converter2 : nesl_utility/PS-Simulink Converter  PhysicalDomain=network_engine_domain  SubClassName=ps_output  LeftPortType=input  RightPortType=output  PseudoPeriodic=off  Frequencies=[]  VectorFormat=1-D array  Unit=rad  AffineConversion=off
  R : PMIOPort  Side=Left
  we : Outport
  theta_e : Outport  Port=2
  wires:
  PS-Simulink Converter1/1 -> Gain/1
  Gain/1 -> we/1
  PS-Simulink Converter2/1 -> Gain3/1
  Constant4/1 -> Math Function1/2
  Gain3/1 -> Math Function1/1
  Math Function1/1 -> theta_e/1
  connections:
  R/RConn1 -- Motion Sensor/LConn1
  Motion Sensor/RConn2 -- PS-Simulink Converter1/LConn1
  MRRef/LConn1 -- Motion Sensor/RConn1
  Motion Sensor/RConn3 -- PS-Simulink Converter2/LConn1

== system FOC_sensored/Mjerenje kuta i brzine3 ==
  Constant4 : Constant  Value=2*pi
  Gain : Gain  Gain=pp
  Gain3 : Gain  Gain=pp
  MRRef : fl_lib/Mechanical/Rotational Elements/Mechanical Rotational Reference
  Math Function1 : Math  Operator=mod
  Motion Sensor : fl_lib/Mechanical/Mechanical Sensors/Ideal Rotational Motion Sensor  reference=foundation.enum.MeasurementReference.difference  acceleration_port=false  velocity_port=true  position_port=true  wrap_angle=simscape.enum.onoff.off  offset=0 deg
  PS-Simulink Converter1 : nesl_utility/PS-Simulink Converter  PhysicalDomain=network_engine_domain  SubClassName=ps_output  LeftPortType=input  RightPortType=output  PseudoPeriodic=off  Frequencies=[]  VectorFormat=1-D array  Unit=rad/s  AffineConversion=off
  PS-Simulink Converter2 : nesl_utility/PS-Simulink Converter  PhysicalDomain=network_engine_domain  SubClassName=ps_output  LeftPortType=input  RightPortType=output  PseudoPeriodic=off  Frequencies=[]  VectorFormat=1-D array  Unit=rad  AffineConversion=off
  R : PMIOPort  Side=Left
  we : Outport
  theta_e : Outport  Port=2
  wires:
  PS-Simulink Converter1/1 -> Gain/1
  Gain/1 -> we/1
  PS-Simulink Converter2/1 -> Gain3/1
  Constant4/1 -> Math Function1/2
  Gain3/1 -> Math Function1/1
  Math Function1/1 -> theta_e/1
  connections:
  R/RConn1 -- Motion Sensor/LConn1
  Motion Sensor/RConn2 -- PS-Simulink Converter1/LConn1
  MRRef/LConn1 -- Motion Sensor/RConn1
  Motion Sensor/RConn3 -- PS-Simulink Converter2/LConn1

== system FOC_sensored/Mjerenje kuta i brzine4 ==
  Constant4 : Constant  Value=2*pi
  Gain : Gain  Gain=pp
  Gain3 : Gain  Gain=pp
  MRRef : fl_lib/Mechanical/Rotational Elements/Mechanical Rotational Reference
  Math Function1 : Math  Operator=mod
  Motion Sensor : fl_lib/Mechanical/Mechanical Sensors/Ideal Rotational Motion Sensor  reference=foundation.enum.MeasurementReference.difference  acceleration_port=false  velocity_port=true  position_port=true  wrap_angle=simscape.enum.onoff.off  offset=0 deg
  PS-Simulink Converter1 : nesl_utility/PS-Simulink Converter  PhysicalDomain=network_engine_domain  SubClassName=ps_output  LeftPortType=input  RightPortType=output  PseudoPeriodic=off  Frequencies=[]  VectorFormat=1-D array  Unit=rad/s  AffineConversion=off
  PS-Simulink Converter2 : nesl_utility/PS-Simulink Converter  PhysicalDomain=network_engine_domain  SubClassName=ps_output  LeftPortType=input  RightPortType=output  PseudoPeriodic=off  Frequencies=[]  VectorFormat=1-D array  Unit=rad  AffineConversion=off
  R : PMIOPort  Side=Left
  we : Outport
  theta_e : Outport  Port=2
  wires:
  PS-Simulink Converter1/1 -> Gain/1
  Gain/1 -> we/1
  PS-Simulink Converter2/1 -> Gain3/1
  Constant4/1 -> Math Function1/2
  Gain3/1 -> Math Function1/1
  Math Function1/1 -> theta_e/1
  connections:
  R/RConn1 -- Motion Sensor/LConn1
  Motion Sensor/RConn2 -- PS-Simulink Converter1/LConn1
  MRRef/LConn1 -- Motion Sensor/RConn1
  Motion Sensor/RConn3 -- PS-Simulink Converter2/LConn1

== system FOC_sensored/Mjerenje kuta i brzine5 ==
  Constant4 : Constant  Value=2*pi
  Gain : Gain  Gain=pp
  Gain3 : Gain  Gain=pp
  MRRef : fl_lib/Mechanical/Rotational Elements/Mechanical Rotational Reference
  Math Function1 : Math  Operator=mod
  Motion Sensor : fl_lib/Mechanical/Mechanical Sensors/Ideal Rotational Motion Sensor  reference=foundation.enum.MeasurementReference.difference  acceleration_port=false  velocity_port=true  position_port=true  wrap_angle=simscape.enum.onoff.off  offset=0 deg
  PS-Simulink Converter1 : nesl_utility/PS-Simulink Converter  PhysicalDomain=network_engine_domain  SubClassName=ps_output  LeftPortType=input  RightPortType=output  PseudoPeriodic=off  Frequencies=[]  VectorFormat=1-D array  Unit=rad/s  AffineConversion=off
  PS-Simulink Converter2 : nesl_utility/PS-Simulink Converter  PhysicalDomain=network_engine_domain  SubClassName=ps_output  LeftPortType=input  RightPortType=output  PseudoPeriodic=off  Frequencies=[]  VectorFormat=1-D array  Unit=rad  AffineConversion=off
  R : PMIOPort  Side=Left
  we : Outport
  theta_e : Outport  Port=2
  wires:
  PS-Simulink Converter1/1 -> Gain/1
  Gain/1 -> we/1
  PS-Simulink Converter2/1 -> Gain3/1
  Constant4/1 -> Math Function1/2
  Gain3/1 -> Math Function1/1
  Math Function1/1 -> theta_e/1
  connections:
  R/RConn1 -- Motion Sensor/LConn1
  Motion Sensor/RConn2 -- PS-Simulink Converter1/LConn1
  MRRef/LConn1 -- Motion Sensor/RConn1
  Motion Sensor/RConn3 -- PS-Simulink Converter2/LConn1

== system FOC_sensored/Mjerenje kuta i brzine6 ==
  Constant4 : Constant  Value=2*pi
  Gain : Gain  Gain=pp
  Gain3 : Gain  Gain=pp
  MRRef : fl_lib/Mechanical/Rotational Elements/Mechanical Rotational Reference
  Math Function1 : Math  Operator=mod
  Motion Sensor : fl_lib/Mechanical/Mechanical Sensors/Ideal Rotational Motion Sensor  reference=foundation.enum.MeasurementReference.difference  acceleration_port=false  velocity_port=true  position_port=true  wrap_angle=simscape.enum.onoff.off  offset=0 deg
  PS-Simulink Converter1 : nesl_utility/PS-Simulink Converter  PhysicalDomain=network_engine_domain  SubClassName=ps_output  LeftPortType=input  RightPortType=output  PseudoPeriodic=off  Frequencies=[]  VectorFormat=1-D array  Unit=rad/s  AffineConversion=off
  PS-Simulink Converter2 : nesl_utility/PS-Simulink Converter  PhysicalDomain=network_engine_domain  SubClassName=ps_output  LeftPortType=input  RightPortType=output  PseudoPeriodic=off  Frequencies=[]  VectorFormat=1-D array  Unit=rad  AffineConversion=off
  R : PMIOPort  Side=Left
  we : Outport
  theta_e : Outport  Port=2
  wires:
  PS-Simulink Converter1/1 -> Gain/1
  Gain/1 -> we/1
  PS-Simulink Converter2/1 -> Gain3/1
  Constant4/1 -> Math Function1/2
  Gain3/1 -> Math Function1/1
  Math Function1/1 -> theta_e/1
  connections:
  R/RConn1 -- Motion Sensor/LConn1
  Motion Sensor/RConn2 -- PS-Simulink Converter1/LConn1
  MRRef/LConn1 -- Motion Sensor/RConn1
  Motion Sensor/RConn3 -- PS-Simulink Converter2/LConn1

== system FOC_sensored/Mjerenje struje1 ==
  Input : Inport
  Current Sensor : ee_lib/Sensors & Transducers/Current Sensor (Three-Phase)  port_option=ee.enum.threePhasePort.composite
  PS-Simulink Converter : nesl_utility/PS-Simulink Converter  PhysicalDomain=network_engine_domain  SubClassName=ps_output  LeftPortType=input  RightPortType=output  PseudoPeriodic=off  Frequencies=[]  VectorFormat=1-D array  Unit=1  AffineConversion=off
  Park Transform : eeTransforms/Park Transform  AxisAlignment=D-axis  PowerInvariant=off
  ~1 : PMIOPort  Side=Left
  ~2 : PMIOPort  Port=2  Side=Right
  Output : Outport
  wires:
  PS-Simulink Converter/1 -> Park Transform/1
  Park Transform/1 -> Output/1
  Input/1 -> Park Transform/2
  connections:
  Current Sensor/LConn1 -- ~1/RConn1
  PS-Simulink Converter/LConn1 -- Current Sensor/RConn1
  Current Sensor/RConn2 -- ~2/RConn1

== system FOC_sensored/Mjerenje struje2 ==
  Input : Inport
  Current Sensor : ee_lib/Sensors & Transducers/Current Sensor (Three-Phase)  port_option=ee.enum.threePhasePort.composite
  PS-Simulink Converter : nesl_utility/PS-Simulink Converter  PhysicalDomain=network_engine_domain  SubClassName=ps_output  LeftPortType=input  RightPortType=output  PseudoPeriodic=off  Frequencies=[]  VectorFormat=1-D array  Unit=1  AffineConversion=off
  Park Transform : eeTransforms/Park Transform  AxisAlignment=D-axis  PowerInvariant=off
  ~1 : PMIOPort  Side=Left
  ~2 : PMIOPort  Port=2  Side=Right
  Output : Outport
  wires:
  PS-Simulink Converter/1 -> Park Transform/1
  Park Transform/1 -> Output/1
  Input/1 -> Park Transform/2
  connections:
  Current Sensor/LConn1 -- ~1/RConn1
  PS-Simulink Converter/LConn1 -- Current Sensor/RConn1
  Current Sensor/RConn2 -- ~2/RConn1

== system FOC_sensored/Mjerenje struje3 ==
  Input : Inport
  Current Sensor : ee_lib/Sensors & Transducers/Current Sensor (Three-Phase)  port_option=ee.enum.threePhasePort.composite
  PS-Simulink Converter : nesl_utility/PS-Simulink Converter  PhysicalDomain=network_engine_domain  SubClassName=ps_output  LeftPortType=input  RightPortType=output  PseudoPeriodic=off  Frequencies=[]  VectorFormat=1-D array  Unit=1  AffineConversion=off
  Park Transform : eeTransforms/Park Transform  AxisAlignment=D-axis  PowerInvariant=off
  ~1 : PMIOPort  Side=Left
  ~2 : PMIOPort  Port=2  Side=Right
  Output : Outport
  wires:
  PS-Simulink Converter/1 -> Park Transform/1
  Park Transform/1 -> Output/1
  Input/1 -> Park Transform/2
  connections:
  Current Sensor/LConn1 -- ~1/RConn1
  PS-Simulink Converter/LConn1 -- Current Sensor/RConn1
  Current Sensor/RConn2 -- ~2/RConn1

== system FOC_sensored/Mjerenje struje4 ==
  Input : Inport
  Current Sensor : ee_lib/Sensors & Transducers/Current Sensor (Three-Phase)  port_option=ee.enum.threePhasePort.composite
  PS-Simulink Converter : nesl_utility/PS-Simulink Converter  PhysicalDomain=network_engine_domain  SubClassName=ps_output  LeftPortType=input  RightPortType=output  PseudoPeriodic=off  Frequencies=[]  VectorFormat=1-D array  Unit=1  AffineConversion=off
  Park Transform : eeTransforms/Park Transform  AxisAlignment=D-axis  PowerInvariant=off
  ~1 : PMIOPort  Side=Left
  ~2 : PMIOPort  Port=2  Side=Right
  Output : Outport
  wires:
  PS-Simulink Converter/1 -> Park Transform/1
  Park Transform/1 -> Output/1
  Input/1 -> Park Transform/2
  connections:
  Current Sensor/LConn1 -- ~1/RConn1
  PS-Simulink Converter/LConn1 -- Current Sensor/RConn1
  Current Sensor/RConn2 -- ~2/RConn1

== system FOC_sensored/Mjerenje struje5 ==
  Input : Inport
  Current Sensor : ee_lib/Sensors & Transducers/Current Sensor (Three-Phase)  port_option=ee.enum.threePhasePort.composite
  PS-Simulink Converter : nesl_utility/PS-Simulink Converter  PhysicalDomain=network_engine_domain  SubClassName=ps_output  LeftPortType=input  RightPortType=output  PseudoPeriodic=off  Frequencies=[]  VectorFormat=1-D array  Unit=1  AffineConversion=off
  Park Transform : eeTransforms/Park Transform  AxisAlignment=D-axis  PowerInvariant=off
  ~1 : PMIOPort  Side=Left
  ~2 : PMIOPort  Port=2  Side=Right
  Output : Outport
  wires:
  PS-Simulink Converter/1 -> Park Transform/1
  Park Transform/1 -> Output/1
  Input/1 -> Park Transform/2
  connections:
  Current Sensor/LConn1 -- ~1/RConn1
  PS-Simulink Converter/LConn1 -- Current Sensor/RConn1
  Current Sensor/RConn2 -- ~2/RConn1

== system FOC_sensored/Mjerenje struje6 ==
  Input : Inport
  Current Sensor : ee_lib/Sensors & Transducers/Current Sensor (Three-Phase)  port_option=ee.enum.threePhasePort.composite
  PS-Simulink Converter : nesl_utility/PS-Simulink Converter  PhysicalDomain=network_engine_domain  SubClassName=ps_output  LeftPortType=input  RightPortType=output  PseudoPeriodic=off  Frequencies=[]  VectorFormat=1-D array  Unit=1  AffineConversion=off
  Park Transform : eeTransforms/Park Transform  AxisAlignment=D-axis  PowerInvariant=off
  ~1 : PMIOPort  Side=Left
  ~2 : PMIOPort  Port=2  Side=Right
  Output : Outport
  wires:
  PS-Simulink Converter/1 -> Park Transform/1
  Park Transform/1 -> Output/1
  Input/1 -> Park Transform/2
  connections:
  Current Sensor/LConn1 -- ~1/RConn1
  PS-Simulink Converter/LConn1 -- Current Sensor/RConn1
  Current Sensor/RConn2 -- ~2/RConn1

== system FOC_sensored/PWM inverter1 ==
  ud_ref : Inport
  uq_ref : Inport  Port=2
  theta_e_mj : Inport  Port=3
  Constant1 : Constant  Value=0  SampleTime=-1
  Gain : Gain
  Gain1 : Gain
  Mux2 : Mux  Inputs=2
  Mux3 : Mux  Inputs=2
  Scope : Scope  NumInputPorts=2
      settings: ActiveDisplayYMinimum=-5.00439749396322  ActiveDisplayYMaximum=16.069405098335697
  Zero-Order Hold1 : ZeroOrderHold  SampleTime=Ts_current
  dq->abc : eeTransforms/Inverse Park Transform  AxisAlignment=D-axis  PowerInvariant=off
  u_abc* : Outport  VectorParamsAs1DForOutWhenUnconnected=off
  wires:
  Constant1/1 -> Mux2/2
  Mux2/1 -> dq->abc/1
  Mux3/1 -> Mux2/1
  theta_e_mj/1 -> dq->abc/2
  dq->abc/1 -> Zero-Order Hold1/1
  ud_ref/1 -> Gain/1
  uq_ref/1 -> Gain1/1
  Gain/1 -> Scope/1, Mux3/1
  Gain1/1 -> Scope/2, Mux3/2
  Zero-Order Hold1/1 -> u_abc*/1

== system FOC_sensored/PWM inverter2 ==
  ud_ref : Inport
  uq_ref : Inport  Port=2
  theta_e_mj : Inport  Port=3
  Constant1 : Constant  Value=0  SampleTime=-1
  Gain : Gain
  Gain1 : Gain
  Mux2 : Mux  Inputs=2
  Mux3 : Mux  Inputs=2
  Scope : Scope  NumInputPorts=2
      settings: ActiveDisplayYMinimum=-5.00439749396322  ActiveDisplayYMaximum=16.069405098335697
  Zero-Order Hold1 : ZeroOrderHold  SampleTime=Ts_current
  dq->abc : eeTransforms/Inverse Park Transform  AxisAlignment=D-axis  PowerInvariant=off
  u_abc* : Outport  VectorParamsAs1DForOutWhenUnconnected=off
  wires:
  Constant1/1 -> Mux2/2
  Mux2/1 -> dq->abc/1
  Mux3/1 -> Mux2/1
  theta_e_mj/1 -> dq->abc/2
  dq->abc/1 -> Zero-Order Hold1/1
  ud_ref/1 -> Gain/1
  uq_ref/1 -> Gain1/1
  Gain/1 -> Scope/1, Mux3/1
  Gain1/1 -> Scope/2, Mux3/2
  Zero-Order Hold1/1 -> u_abc*/1

== system FOC_sensored/PWM inverter3 ==
  ud_ref : Inport
  uq_ref : Inport  Port=2
  theta_e_mj : Inport  Port=3
  Constant1 : Constant  Value=0  SampleTime=-1
  Gain : Gain
  Gain1 : Gain
  Mux2 : Mux  Inputs=2
  Mux3 : Mux  Inputs=2
  Scope : Scope  NumInputPorts=2
      settings: ActiveDisplayYMinimum=-5.00439749396322  ActiveDisplayYMaximum=16.069405098335697
  Zero-Order Hold1 : ZeroOrderHold  SampleTime=Ts_current
  dq->abc : eeTransforms/Inverse Park Transform  AxisAlignment=D-axis  PowerInvariant=off
  u_abc* : Outport  VectorParamsAs1DForOutWhenUnconnected=off
  wires:
  Constant1/1 -> Mux2/2
  Mux2/1 -> dq->abc/1
  Mux3/1 -> Mux2/1
  theta_e_mj/1 -> dq->abc/2
  dq->abc/1 -> Zero-Order Hold1/1
  ud_ref/1 -> Gain/1
  uq_ref/1 -> Gain1/1
  Gain/1 -> Scope/1, Mux3/1
  Gain1/1 -> Scope/2, Mux3/2
  Zero-Order Hold1/1 -> u_abc*/1

== system FOC_sensored/PWM inverter4 ==
  ud_ref : Inport
  uq_ref : Inport  Port=2
  theta_e_mj : Inport  Port=3
  Constant1 : Constant  Value=0  SampleTime=-1
  Gain : Gain
  Gain1 : Gain
  Mux2 : Mux  Inputs=2
  Mux3 : Mux  Inputs=2
  Scope : Scope  NumInputPorts=2
      settings: ActiveDisplayYMinimum=-5.00439749396322  ActiveDisplayYMaximum=16.069405098335697
  Zero-Order Hold1 : ZeroOrderHold  SampleTime=Ts_current
  dq->abc : eeTransforms/Inverse Park Transform  AxisAlignment=D-axis  PowerInvariant=off
  u_abc* : Outport  VectorParamsAs1DForOutWhenUnconnected=off
  wires:
  Constant1/1 -> Mux2/2
  Mux2/1 -> dq->abc/1
  Mux3/1 -> Mux2/1
  theta_e_mj/1 -> dq->abc/2
  dq->abc/1 -> Zero-Order Hold1/1
  ud_ref/1 -> Gain/1
  uq_ref/1 -> Gain1/1
  Gain/1 -> Scope/1, Mux3/1
  Gain1/1 -> Scope/2, Mux3/2
  Zero-Order Hold1/1 -> u_abc*/1

== system FOC_sensored/PWM inverter5 ==
  ud_ref : Inport
  uq_ref : Inport  Port=2
  theta_e_mj : Inport  Port=3
  Constant1 : Constant  Value=0  SampleTime=-1
  Gain : Gain
  Gain1 : Gain
  Mux2 : Mux  Inputs=2
  Mux3 : Mux  Inputs=2
  Scope : Scope  NumInputPorts=2
      settings: ActiveDisplayYMinimum=-5.00439749396322  ActiveDisplayYMaximum=16.069405098335697
  Zero-Order Hold1 : ZeroOrderHold  SampleTime=Ts_current
  dq->abc : eeTransforms/Inverse Park Transform  AxisAlignment=D-axis  PowerInvariant=off
  u_abc* : Outport  VectorParamsAs1DForOutWhenUnconnected=off
  wires:
  Constant1/1 -> Mux2/2
  Mux2/1 -> dq->abc/1
  Mux3/1 -> Mux2/1
  theta_e_mj/1 -> dq->abc/2
  dq->abc/1 -> Zero-Order Hold1/1
  ud_ref/1 -> Gain/1
  uq_ref/1 -> Gain1/1
  Gain/1 -> Scope/1, Mux3/1
  Gain1/1 -> Scope/2, Mux3/2
  Zero-Order Hold1/1 -> u_abc*/1
